simulink model "Ex309"  (R2021b)
settings: Solver=VariableStepAuto  StartTime=0.0  StopTime=10.0  RelTol=1e-3
settings Model: Creator=abdul  LastModifiedBy=abdul

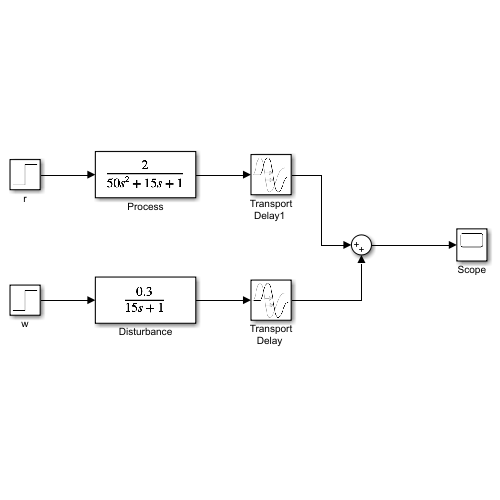
[thumbnail: Simulink's stored preview of the top-level diagram]
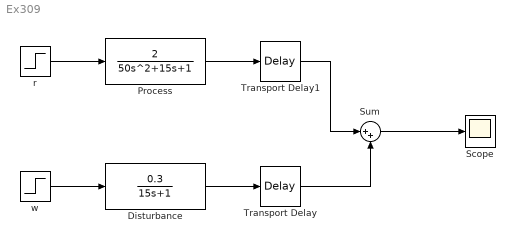
== system Ex309 ==
  " Scope " : Scope
  Disturbance : TransferFcn  Numerator=[0.3]  Denominator=[15 1]
  Process : TransferFcn  Numerator=[2]  Denominator=[50 15 1]
  Sum : Sum  Inputs=|++
  "Transport Delay " : TransportDelay  DelayTime=5
  "Transport Delay1 " : TransportDelay  DelayTime=5
  r : Step  SampleTime=0
  w : Step  SampleTime=0
  wires:
  Process/1 -> "Transport Delay1 "/1
  Disturbance/1 -> "Transport Delay "/1
  w/1 -> Disturbance/1
  r/1 -> Process/1
  "Transport Delay1 "/1 -> Sum/1
  "Transport Delay "/1 -> Sum/2
  Sum/1 -> " Scope "/1
